simulink model "p2"  (R2021a)
settings: Solver=VariableStepAuto  StartTime=0.0  StopTime=inf  FixedStep=1  RelTol=1e-3
settings Model: Creator=Abbas  LastModifiedBy=Abbas
settings SolverCC: ZeroCrossAlgorithm=Adaptive
settings DebuggingCC: IgnoredZcDiagnostic=none

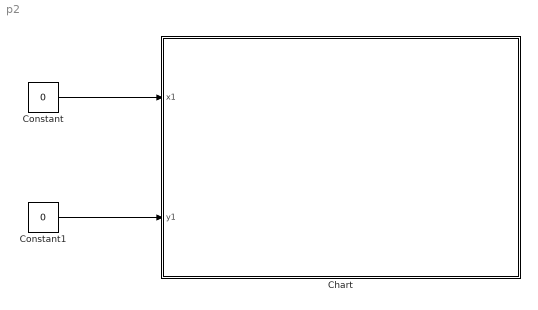
== system p2 ==
  Chart : Stateflow chart  TreatAsAtomicUnit=on
  Constant : Constant  Value=0
  Constant1 : Constant  Value=0
  wires:
  Constant/1 -> Chart/1(x1)
  Constant1/1 -> Chart/2(y1)

== stateflow chart p2/Chart ==
  settings: updateMethod=CONTINUOUS
  state UP
    du:
    y0_dot=v_y;
  state RIGHT
    du:
    x0_dot =v_x;
  state STOP
    du:
    x0_dot=0;
    y0_dot=0;
  state DIRECT
    du:
    x0_dot=sin(atan(a))*(v_d)*(x1-x0)/abs(x1-x0);
    y0_dot=cos(atan(a))*(v_d)*(x1-x0)/abs(x1-x0);
  state DOWN
    du:
    y0_dot= - v_y;
  state LEFT
    du:
    x0_dot=-v_x;
  UP -> STOP [order 1] : [(abs(y1-y0) > 0.9) & after(0.1,sec)]
  UP -> STOP [order 2] : [(abs(y1-y0) < 0.9) & after(0.1,sec)]{y0 = y1;}
  STOP -> UP [order 2] : [y1>y0 &  ((((x1-x0)^2 + (y1-y0)^2)/25) >  ((abs(x1-x0)/6 + abs(y1-y0)/8))^2) ]
  STOP -> RIGHT [order 4] : [y1>=y0 & x1>x0]
  RIGHT -> STOP [order 1] : [(abs(x1-x0) < 0.7) & after(0.1,sec)]{x0=x1;}
  RIGHT -> STOP [order 2] : [(abs(x1-x0) > 0.7) & after(0.1,sec)]
  (default) -> STOP : {x0 = 100;  y0 = 0;}
  STOP -> STOP [order 5] : [[x1==x0 & y1==y0]]
  DIRECT -> STOP [order 1] : [(abs(x1-x0)>0.7) & (abs(y1-y0)>0.9)  & after (0.1,sec)]
  DIRECT -> STOP [order 2] : [(abs(x1-x0)<=0.7) & (abs(y1-y0)>0.9)  & after (0.1,sec)]{x0=x1;}
  DIRECT -> STOP [order 3] : [(abs(x1-x0)>0.7) & (abs(y1-y0)<=0.9)  & after (0.1,sec)]{y0=y1;}
  DIRECT -> STOP [order 4] : [(abs(x1-x0)<=0.7) & (abs(y1-y0)<=0.9)  & after (0.1,sec)]{y0=y1;x0=x1;}
  STOP -> DIRECT [order 3] : [ (x1~=x0 & y1~=y0) &((((x1-x0)^2 + (y1-y0)^2)/25) <=  ((abs(x1-x0)/6 + abs(y1-y0)/8))^2)  ]{a=(y1-y0)/(x1-x0)}
  DOWN -> STOP [order 2] : [(abs(y1-y0) < 0.9) & after(0.1,sec)]{y0 = y1;}
  STOP -> DOWN [order 1] : [y1<y0 &  ((((x1-x0)^2 + (y1-y0)^2)/25) >  ((abs(x1-x0)/6 + abs(y1-y0)/8))^2)]
  DOWN -> STOP [order 1] : [(abs(y1-y0) > 0.9) & after(0.1,sec)]
  LEFT -> STOP [order 2] : [(abs(x1-x0) > 0.7) & after(0.1,sec)]
  LEFT -> STOP [order 1] : [(abs(x1-x0) < 0.7) & after(0.1,sec)]{x0=x1;}
  STOP -> LEFT [order 6] : [y1==y0 & x1<x0]
  data: x0 local; y0 local; x1 input; y1 input; v_x constant double =6; v_y constant double =8; v_d constant double =5; a local
  data x0 settings: updateMethod=SF_CONTINUOUS_TIME_DATA
  data y0 settings: updateMethod=SF_CONTINUOUS_TIME_DATA
